simulink model "sistemaNonLineare_disturbi"  (R2023b)
settings: Solver=VariableStepAuto  StartTime=0.0  StopTime=5  RelTol=1e-3
undefined symbols (not defined in the file): C, u_e, x_e, ze
libraries: simulink x2, cstblocks x1
settings Model: Creator=Utente  LastModifiedBy=Utente

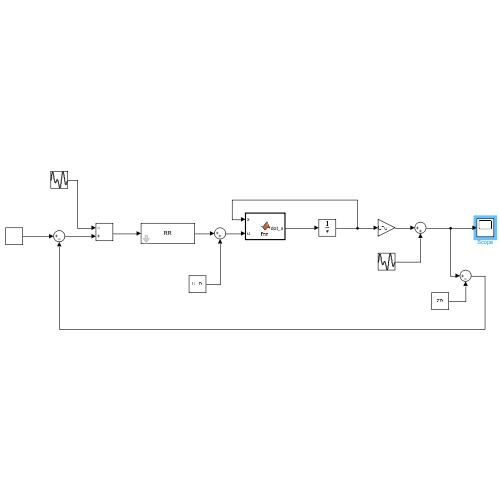
[thumbnail: Simulink's stored preview of the top-level diagram]
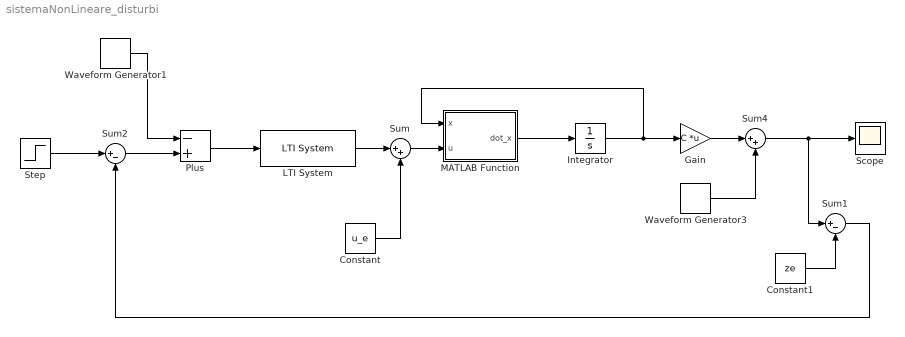
== system sistemaNonLineare_disturbi ==
  Constant : Constant  Value=u_e
  Constant1 : Constant  Value=ze
  Gain : Gain  Gain=C  Multiplication=Matrix(K*u)
  Integrator : Integrator  InitialCondition=x_e
  LTI System : cstblocks/LTI System  sys=RR  IC=[]  PadeOrder=0
  MATLAB Function : MATLAB Function  TreatAsAtomicUnit=on
  Plus : Sum  Inputs=-+
  Scope : Scope
  Step : Step  SampleTime=0
  Sum : Sum  Inputs=|++
  Sum1 : Sum  Inputs=|+-
  Sum2 : Sum  Inputs=|+-
  Sum4 : Sum  Inputs=|++
  Waveform Generator1 : simulink/Sources/Waveform Generator  OutMin=[]  OutMax=[]  OutDataTypeStr=double  SelectedSignal=1  Signals=sin(0.2, 80000, 0) + sin(0.2, 160000, 0) + sin(0.2, 240000, 0) + sin(0.2, 320000, 0)  BlockNames=MultiportSwitch_4a0dc30300f5477  SampleTime=5e-6
  Waveform Generator3 : simulink/Sources/Waveform Generator  OutMin=[]  OutMax=[]  OutDataTypeStr=double  SelectedSignal=1  Signals=sin(1, 0.01, 0)+sin(1, 2*0.01, 0)+sin(1, 3*0.01, 0)+sin(1, 4*0.01, 0)  BlockNames=MultiportSwitch_ef3f03ef5be8455  SampleTime=5e-3
  wires:
  LTI System/1 -> Sum/1
  Constant/1 -> Sum/2
  Sum/1 -> MATLAB Function/2(u)
  MATLAB Function/1(dot_x) -> Integrator/1
  Integrator/1 -> MATLAB Function/1(x), Gain/1
  Sum4/1 -> Sum1/1, Scope/1
  Constant1/1 -> Sum1/2
  Step/1 -> Sum2/1
  Gain/1 -> Sum4/1
  Waveform Generator3/1 -> Sum4/2
  Waveform Generator1/1 -> Plus/1
  Sum2/1 -> Plus/2
  Sum1/1 -> Sum2/2
  Plus/1 -> LTI System/1

== matlab function sistemaNonLineare_disturbi/MATLAB Function ==
  data: x input; u input; dot_x output
function dot_x = fcn(x,u)

m = 2500;       %% mass
b = 350;        %% smorzamento
k = 5*10^5;     %% cost. elastica lineare
n = 3;
g = 9.81;
beta = 0.1;

dot_x = zeros(2,1);

dot_x(1) = x(2);

dot_x(2) = -g - b*x(2)/m - k*x(1)/m  + beta/m * (x(2)^3 + n*x(2)*sin(n*x(2))^2) + u/m;
